simulink model "Template"  (Simulink 7.3)
settings: Solver=ode45  StartTime=0.0  StopTime=10.0  RelTol=1e-3
undefined symbols (not defined in the file): eta1_0_real, v1_0_real, velocitySatValues1
libraries: dspmtrx3 x21, simulink x14, dspindex x5, marine_gnc x4, simulink_extras x1, dspinverses x1
(part 2 of 4)

== system Template/Main Subsystems/Control/LgV2/alpha^q ==
  Add : Sum  OutDataType=fixdt(1, 16)  OutScaling=2^-10
  Add2 : Sum  OutDataType=fixdt(1, 16)  OutScaling=2^-10
  Add3 : Sum  OutDataType=fixdt(1, 16)  OutScaling=2^-10
  I : dspmtrx3/Constant Diagonal Matrix  SystemSampleTime=-1  q=[1 1 1 ]  frame=off  dataType=Inherit from 'Constant(s) along diagonal'  isSigned=on  wordLen=16  udDataType=sfix(16)  fracBitsMode=Best precision  numFracBits=15
  Product1 : Product  OutDataType=fixdt(1, 16)  OutScaling=2^0  RndMeth=Zero
  Product3 : Product  Inputs=3  Multiplication=Matrix(*)  OutDataType=fixdt(1, 16)  OutScaling=2^0  RndMeth=Zero
  Product4 : Product  Multiplication=Matrix(*)  OutDataType=fixdt(1, 16)  OutScaling=2^0  RndMeth=Zero
  tag scope: alpha__q=global
  wires:
  Add3/1 -> [alpha__q]
  Product1/1 -> Add/2
  [LgV2_kappa_1] -> Product1/1
  I/1 -> Product1/2
  Add/1 -> Product3/1
  Add2/1 -> Product4/2
  [R_psi__T] -> Product3/2, Product4/1
  [chi__q] -> Product3/3
  Product3/1 -> Add3/1
  Product4/1 -> Add3/2
  [LgV2_K_p] -> Add/1
  [g_q__q] -> Add2/1
  [g_s__q] -> Add2/2

== system Template/Main Subsystems/Control/LgV2/alpha^s ==
  Add1 : Sum  OutDataType=fixdt(1, 16)  OutScaling=2^-10
  Add2 : Sum  OutDataType=fixdt(1, 16)  OutScaling=2^-10
  Add3 : Sum  OutDataType=fixdt(1, 16)  OutScaling=2^-10
  I : dspmtrx3/Constant Diagonal Matrix  SystemSampleTime=-1  q=[1 1 1 ]  frame=off  dataType=Inherit from 'Constant(s) along diagonal'  isSigned=on  wordLen=16  udDataType=sfix(16)  fracBitsMode=Best precision  numFracBits=15
  Product1 : Product  OutDataType=fixdt(1, 16)  OutScaling=2^0  RndMeth=Zero
  Product3 : Product  Inputs=3  Multiplication=Matrix(*)  OutDataType=fixdt(1, 16)  OutScaling=2^0  RndMeth=Zero
  Product4 : Product  Multiplication=Matrix(*)  OutDataType=fixdt(1, 16)  OutScaling=2^0  RndMeth=Zero
  tag scope: alpha__s=global
  wires:
  Add3/1 -> [alpha__s]
  Product1/1 -> Add1/2
  [LgV2_kappa_1] -> Product1/1
  I/1 -> Product1/2
  Add1/1 -> Product3/1
  Add2/1 -> Product4/2
  [R_psi__T] -> Product3/2, Product4/1
  [chi__s] -> Product3/3
  Product3/1 -> Add3/1
  Product4/1 -> Add3/2
  [LgV2_K_p] -> Add1/1
  [g_q__s] -> Add2/1
  [g_s__s] -> Add2/2

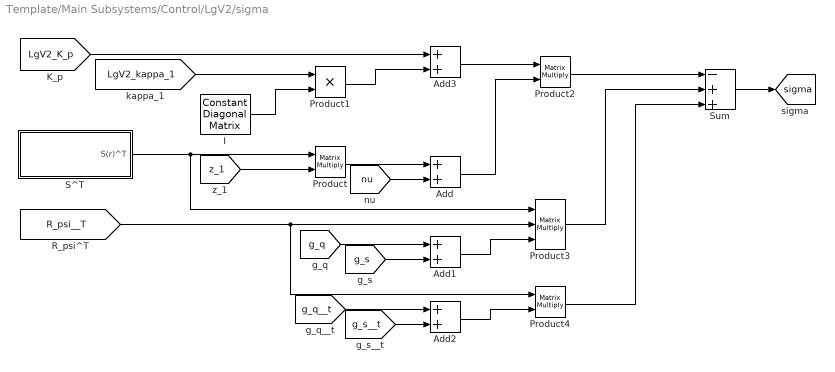
== system Template/Main Subsystems/Control/LgV2/sigma ==
  Add{,1..3} (4 alike) : Sum  OutDataType=fixdt(1, 16)  OutScaling=2^-10
  I : dspmtrx3/Constant Diagonal Matrix  SystemSampleTime=-1  q=[1 1 1 ]  frame=off  dataType=Inherit from 'Constant(s) along diagonal'  isSigned=on  wordLen=16  udDataType=sfix(16)  fracBitsMode=Best precision  numFracBits=15
  Product : Product  Multiplication=Matrix(*)  OutDataType=fixdt(1, 16)  OutScaling=2^0  RndMeth=Zero
  Product1 : Product  OutDataType=fixdt(1, 16)  OutScaling=2^0  RndMeth=Zero
  Product2 : Product  Multiplication=Matrix(*)  OutDataType=fixdt(1, 16)  OutScaling=2^0  RndMeth=Zero
  Product3 : Product  Inputs=3  Multiplication=Matrix(*)  OutDataType=fixdt(1, 16)  OutScaling=2^0  RndMeth=Zero
  Product4 : Product  Multiplication=Matrix(*)  OutDataType=fixdt(1, 16)  OutScaling=2^0  RndMeth=Zero
  S^T : Subsystem
  Sum : Sum  Inputs=-++  OutDataType=fixdt(1, 16)  OutScaling=2^-10
  tag scope: sigma=global
  wires:
  Sum/1 -> [sigma]
  [LgV2_K_p] -> Add3/1
  Product1/1 -> Add3/2
  [LgV2_kappa_1] -> Product1/1
  I/1 -> Product1/2
  S^T/1(S(r)^T) -> Product/1, Product3/1
  [z_1] -> Product/2
  Product/1 -> Add/1
  [nu] -> Add/2
  Add3/1 -> Product2/1
  Add/1 -> Product2/2
  Product2/1 -> Sum/1
  [g_q] -> Add1/1
  [g_s] -> Add1/2
  [g_q__t] -> Add2/1
  [g_s__t] -> Add2/2
  [R_psi__T] -> Product3/2, Product4/1
  Add1/1 -> Product3/3
  Add2/1 -> Product4/2
  Product3/1 -> Sum/2
  Product4/1 -> Sum/3

== system Template/Main Subsystems/Control/LgV2/z_1 ==
  Heading to -pi/pi : Subsystem
  Heading to -pi/pi1 : Subsystem
  Product : Product  Multiplication=Matrix(*)  OutDataType=fixdt(1, 16)  OutScaling=2^0  RndMeth=Zero
  Subtract : Sum  Inputs=+-  OutDataType=fixdt(1, 16)  OutScaling=2^-10
  tag scope: z_1=global
  wires:
  Subtract/1 -> Heading to -pi/pi1/1(eta(3) [0 2pi])
  Product/1 -> [z_1]
  Heading to -pi/pi/1(eta(3) [-pi pi]) -> Subtract/1
  Heading to -pi/pi1/1(eta(3) [-pi pi]) -> Product/2
  [R_psi__T] -> Product/1
  [chi] -> Subtract/2
  [eta] -> Heading to -pi/pi/1(eta(3) [0 2pi])

== system Template/Main Subsystems/Control/LgV2/z_2 ==
  Subtract : Sum  Inputs=+-  OutDataType=fixdt(1, 16)  OutScaling=2^-10
  tag scope: z_2=global
  wires:
  [alpha] -> Subtract/2
  Subtract/1 -> [z_2]
  [nu] -> Subtract/1

== system Template/Main Subsystems/Control/LgV2/zeta ==
  Integrator : Integrator  InitialCondition=[0 0 0]'
  Product : Product  Multiplication=Matrix(*)  OutDataType=fixdt(1, 16)  OutScaling=2^0  RndMeth=Zero
  tag scope: zeta=global
  wires:
  [R_psi] -> Product/1
  [z_2] -> Product/2
  Integrator/1 -> [zeta]
  Product/1 -> Integrator/1

== system Template/Main Subsystems/Control/Thruster allocation/VSP030 BT040 ==
  f_act : Inport
  BT_power_limit : Constant  Value=0.4
  Mux1 : Mux  Inputs=3
  VSP_speeds : Constant  Value=0.3
  f_act to u_act : Subsystem
  TC : Outport  OutDataType=fixdt(1, 16)  OutScaling=2^0
  wires:
  Mux1/1 -> TC/1
  f_act/1 -> f_act to u_act/1(f_act)
  BT_power_limit/1 -> Mux1/2
  VSP_speeds/1 -> Mux1/3
  f_act to u_act/1(u_act) -> Mux1/1

== system Template/Main Subsystems/Control/Thruster allocation/tau to f_act ==
  tau : Inport
  Product : Product  Multiplication=Matrix(*)  OutDataType=fixdt(1, 16)  OutScaling=2^0  RndMeth=Zero
  Pseudoinverse : dspinverses/Pseudoinverse  wanterr=off
  f_act : Outport
  wires:
  [B] -> Pseudoinverse/1
  Pseudoinverse/1 -> Product/1
  tau/1 -> Product/2
  Product/1 -> f_act/1

== system Template/Main Subsystems/Guidance/Line-Of-Sight Path-Following/Heading ==
  Demux : Demux  Outputs=2
  Demux1 : Demux  Outputs=2
  Demux2 : Demux  Outputs=2
  psi_d eq : Subsystem
  psi_d^s eq : Subsystem
  psi_d^s^2 eq : Subsystem
  tag scope: psi_d=global, psi_d__s=global, psi_d__s__2=global
  wires:
  psi_d^s eq/3(den) -> psi_d^s^2 eq/2(den)
  psi_d^s eq/2(num) -> psi_d^s^2 eq/1(num)
  Demux2/2 -> psi_d^s^2 eq/8(y_d^s^3)
  Demux2/1 -> psi_d^s^2 eq/7(x_d^s^3)
  psi_d^s^2 eq/1(psi_d^s^2) -> [psi_d__s__2]
  [p_d__s__3] -> Demux2/1
  psi_d^s eq/1(psi_d^s) -> [psi_d__s]
  Demux1/2 -> psi_d^s^2 eq/6(y_d^s^2), psi_d^s eq/4(y_d^s^2)
  Demux1/1 -> psi_d^s^2 eq/5(x_d^s^2), psi_d^s eq/3(x_d^s^2)
  [p_d__s__2] -> Demux1/1
  [p_d__s] -> Demux/1
  Demux/2 -> psi_d^s^2 eq/4(y_d^s), psi_d^s eq/2(y_d^s), psi_d eq/2(y_d^s)
  Demux/1 -> psi_d^s^2 eq/3(x_d^s), psi_d^s eq/1(x_d^s), psi_d eq/1(x_d^s)
  psi_d eq/1(psi_d) -> [psi_d]

== system Template/Main Subsystems/Guidance/Line-Of-Sight Path-Following/Line-Of-Sight ==
  Dynamic LOS assigment for qdot : Subsystem
  Dynamic assigment for sdot : Subsystem
  Gradient update law for sdot : Subsystem
  LOS heading : Subsystem
  Position error signals : Subsystem
  Subtract : Sum  Inputs=+-  OutDataType=fixdt(1, 16)  OutScaling=2^-10
  Virtual Vessel : Subsystem
  tag scope: diff_q_p_d=global
  wires:
  Gradient update law for sdot/3(omega_s^s) -> Dynamic assigment for sdot/6(omega_s^s)
  Gradient update law for sdot/2(omega_s^q) -> Dynamic assigment for sdot/5(omega_s^q)
  Position error signals/4(epsilon_n^q) -> Dynamic assigment for sdot/1(epsilon_n^q), LOS heading/4(epsilon_n^q)
  Position error signals/3(epsilon_n^s^2) -> LOS heading/3(epsilon_n^s^2)
  Position error signals/2(epsilon_n^q^2) -> LOS heading/2(epsilon_n^q^2)
  Position error signals/1(epsilon_n^qs) -> LOS heading/1(epsilon_n^qs)
  Position error signals/5(epsilon_n^s) -> Dynamic assigment for sdot/2(epsilon_n^s), LOS heading/5(epsilon_n^s)
  Position error signals/6(epsilon_n) -> LOS heading/6(epsilon_n), Dynamic assigment for sdot/3(epsilon_n)
  Gradient update law for sdot/1(omega_s) -> Dynamic assigment for sdot/4(omega_s)
  Subtract/1 -> [diff_q_p_d]
  [q] -> Subtract/1
  [p_d] -> Subtract/2

== system Template/Main Subsystems/Guidance/Line-Of-Sight Path-Following/Path ==
  note: Path Selector == 1: Linear path
      | Path Selector == 0: Ellipse path
  Ellipse path : Subsystem
  Path Switch workaround + limiter : Subsystem
  Straight path : Subsystem

== system Template/Main Subsystems/Guidance/Line-Of-Sight Path-Following/Speed assigment ==
  Derivative : Derivative
  v_s eq : Subsystem
  v_s^s eq : Subsystem
  v_s^t eq : Subsystem
  tag scope: u_d__t=global, v_s=global, v_s__s=global, v_s__t=global
  wires:
  Derivative/1 -> v_s^t eq/2(u_d^t), [u_d__t]
  v_s^t eq/1(v_s^t) -> [v_s__t]
  [p_d__s__2] -> v_s^s eq/4(p_d^s^2)
  [p_d__s] -> v_s^s eq/3(p_d^s)
  v_s^s eq/1(v_s^s) -> [v_s__s]
  [u_d] -> Derivative/1, v_s^s eq/2(u_d), v_s eq/2(u_d)
  [abs_p_d__s] -> v_s eq/1(|p_d^s|), v_s^s eq/1(|p_d^s|), v_s^t eq/1(|p_d^s|)
  v_s eq/1(v_s) -> [v_s]

== system Template/Main Subsystems/Plant/CSE1/Bow Thruster ==
  Bow Thruster Direction u_5 : Inport
  Bow Thruster Power : Inport  Port=2
  Add : Sum  Inputs=+++
  BT_D_Gain1 : Gain  Gain=0.02
  BT_D_Gain2 : Gain  Gain=0.02
  BT_L_Gain1 : Gain  Gain=0.02
  BT_L_Gain2 : Gain  Gain=-0.02
  BT_Power_Offset1 : Constant  Value=0.05
  BT_Power_Offset2 : Constant  Value=0.05
  BT_Power_Offset3 : Constant  Value=0.05
  Constant : Constant  Value=0  OutDataType=fixdt(1, 16)  OutScaling=2^0
  Constant1 : Constant  Value=0  OutDataType=fixdt(1, 16)  OutScaling=2^0
  Neg : Gain  Gain=-1  ParameterDataType=fixdt(1, 16)  ParameterScaling=2^0  OutDataType=fixdt(1, 16)  OutScaling=2^0
  SIT PWM0 BT : S-Function  Priority=1  FunctionName=NI_SIT_IO  Parameters=width dtype portnum stime stype btype  EnableBusSupport=off  mask(SIT Outport){portnum=1, width=-1, stime=-1, dtype=auto, stype=auto, btype=0}
      mask prompts: portnum "Port number:"; width "Port dimensions (-1 for dynamically sized):"; stime "Sample time (-1 for inherited):"; dtype "Data type:"; stype "Signal type:"; btype "Block type:"
      mask help: Use this outport on any level of nested subsystems to allow the LabVIEW Simulation Interface Toolkit to map hardware to it.
      mask init:
      | NI_SIT_IO_init;
      settings: CopyFcn=NI_SIT_IO_callbacks(1);  DeleteFcn=NI_SIT_IO_callbacks(2);
      mask StyleString: edit,edit,edit,popup(auto|double|single|int8|uint8|int16|uint16|int32|uint32|boolean),popup(auto|real|complex),edit
      mask CallbackString: NI_SIT_IO_callbacks(3);|||NI_SIT_IO_callbacks(4);||
      mask TabNameString: Parameters,Parameters,Parameters,Parameters,Parameters,Parameters
      mask Display:
      | patch([-x x], [-y y], [.90980 .81960 .32156]);
      | plot([0 -x x 0], [rad -y y rad]);
      | fprintf('SIT%d', portnum);
  Saturation Dynamic : simulink/Discontinuities/Saturation Dynamic  SystemSampleTime=-1  OutMin=[]  OutMax=[]  OutDataTypeStr=Inherit: Same as second input  OutDataType=fixdt(1, 16)  OutScaling=2^-10  DoSatur=off
  Saturation Dynamic1 : simulink/Discontinuities/Saturation Dynamic  SystemSampleTime=-1  OutMin=[]  OutMax=[]  OutDataTypeStr=Inherit: Same as second input  OutDataType=fixdt(1, 16)  OutScaling=2^-10  DoSatur=off
  Saturation Dynamic2 : simulink/Discontinuities/Saturation Dynamic  SystemSampleTime=-1  OutMin=[]  OutMax=[]  OutDataTypeStr=Inherit: Same as second input  OutDataType=fixdt(1, 16)  OutScaling=2^-10  DoSatur=off
  Sum1 : Sum  Inputs=|++
  Sum2 : Sum  Inputs=|++
  Terminator : Terminator
  Terminator1 : Terminator
  wires:
  Bow Thruster Direction u_5/1 -> BT_D_Gain1/1, Saturation Dynamic1/2, BT_D_Gain2/1, Saturation Dynamic2/2
  BT_D_Gain1/1 -> Add/1
  BT_D_Gain2/1 -> Add/3
  BT_Power_Offset1/1 -> Add/2
  Add/1 -> Saturation Dynamic/2
  Bow Thruster Power/1 -> BT_L_Gain2/1, Saturation Dynamic2/1, BT_L_Gain1/1, Neg/1
  Sum1/1 -> Saturation Dynamic/1
  BT_L_Gain1/1 -> Sum1/1
  BT_L_Gain2/1 -> Sum2/1
  Sum2/1 -> Saturation Dynamic/3
  BT_Power_Offset2/1 -> Sum1/2
  BT_Power_Offset3/1 -> Sum2/2
  Saturation Dynamic/1 -> SIT PWM0 BT/1
  Saturation Dynamic2/1 -> Terminator1/1
  Saturation Dynamic1/1 -> Terminator/1
  Constant/1 -> Saturation Dynamic1/1
  Constant1/1 -> Saturation Dynamic2/3
  Neg/1 -> Saturation Dynamic1/3

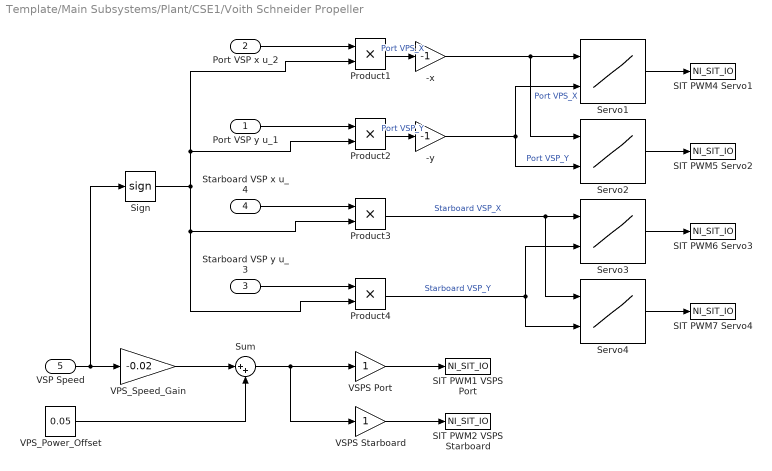
== system Template/Main Subsystems/Plant/CSE1/Voith Schneider Propeller  ==
  Port VSP y u_1 : Inport
  Port VSP x u_2 : Inport  Port=2
  Starboard VSP y u_3 : Inport  Port=3
  Starboard VSP x u_4 : Inport  Port=4
  VSP Speed : Inport  Port=5
  -x : Gain  Gain=-1
  -y : Gain  Gain=-1
  Product{1..4} (4 alike) : Product  RndMeth=Zero
  SIT PWM1 VSPS Port : S-Function  Priority=5  FunctionName=NI_SIT_IO  Parameters=width dtype portnum stime stype btype  EnableBusSupport=off  mask(SIT Outport){portnum=5, width=-1, stime=-1, dtype=auto, stype=auto, btype=0}
      mask prompts: portnum "Port number:"; width "Port dimensions (-1 for dynamically sized):"; stime "Sample time (-1 for inherited):"; dtype "Data type:"; stype "Signal type:"; btype "Block type:"
      mask help: Use this outport on any level of nested subsystems to allow the LabVIEW Simulation Interface Toolkit to map hardware to it.
      mask init:
      | NI_SIT_IO_init;
      settings: CopyFcn=NI_SIT_IO_callbacks(1);  DeleteFcn=NI_SIT_IO_callbacks(2);
      mask StyleString: edit,edit,edit,popup(auto|double|single|int8|uint8|int16|uint16|int32|uint32|boolean),popup(auto|real|complex),edit
      mask CallbackString: NI_SIT_IO_callbacks(3);|||NI_SIT_IO_callbacks(4);||
      mask TabNameString: Parameters,Parameters,Parameters,Parameters,Parameters,Parameters
      mask Display:
      | patch([-x x], [-y y], [.90980 .81960 .32156]);
      | plot([0 -x x 0], [rad -y y rad]);
      | fprintf('SIT%d', portnum);
  SIT PWM2 VSPS Starboard : S-Function  Priority=6  FunctionName=NI_SIT_IO  Parameters=width dtype portnum stime stype btype  EnableBusSupport=off  mask(SIT Outport){portnum=6, width=-1, stime=-1, dtype=auto, stype=auto, btype=0}
      mask prompts: portnum "Port number:"; width "Port dimensions (-1 for dynamically sized):"; stime "Sample time (-1 for inherited):"; dtype "Data type:"; stype "Signal type:"; btype "Block type:"
      mask help: Use this outport on any level of nested subsystems to allow the LabVIEW Simulation Interface Toolkit to map hardware to it.
      mask init:
      | NI_SIT_IO_init;
      settings: CopyFcn=NI_SIT_IO_callbacks(1);  DeleteFcn=NI_SIT_IO_callbacks(2);
      mask StyleString: edit,edit,edit,popup(auto|double|single|int8|uint8|int16|uint16|int32|uint32|boolean),popup(auto|real|complex),edit
      mask CallbackString: NI_SIT_IO_callbacks(3);|||NI_SIT_IO_callbacks(4);||
      mask TabNameString: Parameters,Parameters,Parameters,Parameters,Parameters,Parameters
      mask Display:
      | patch([-x x], [-y y], [.90980 .81960 .32156]);
      | plot([0 -x x 0], [rad -y y rad]);
      | fprintf('SIT%d', portnum);
  SIT PWM4 Servo1 : S-Function  Priority=1  FunctionName=NI_SIT_IO  Parameters=width dtype portnum stime stype btype  EnableBusSupport=off  mask(SIT Outport){portnum=1, width=-1, stime=-1, dtype=auto, stype=auto, btype=0}
      mask prompts: portnum "Port number:"; width "Port dimensions (-1 for dynamically sized):"; stime "Sample time (-1 for inherited):"; dtype "Data type:"; stype "Signal type:"; btype "Block type:"
      mask help: Use this outport on any level of nested subsystems to allow the LabVIEW Simulation Interface Toolkit to map hardware to it.
      mask init:
      | NI_SIT_IO_init;
      settings: CopyFcn=NI_SIT_IO_callbacks(1);  DeleteFcn=NI_SIT_IO_callbacks(2);
      mask StyleString: edit,edit,edit,popup(auto|double|single|int8|uint8|int16|uint16|int32|uint32|boolean),popup(auto|real|complex),edit
      mask CallbackString: NI_SIT_IO_callbacks(3);|||NI_SIT_IO_callbacks(4);||
      mask TabNameString: Parameters,Parameters,Parameters,Parameters,Parameters,Parameters
      mask Display:
      | patch([-x x], [-y y], [.90980 .81960 .32156]);
      | plot([0 -x x 0], [rad -y y rad]);
      | fprintf('SIT%d', portnum);
  SIT PWM5 Servo2 : S-Function  Priority=2  FunctionName=NI_SIT_IO  Parameters=width dtype portnum stime stype btype  EnableBusSupport=off  mask(SIT Outport){portnum=2, width=-1, stime=-1, dtype=auto, stype=auto, btype=0}
      mask prompts: portnum "Port number:"; width "Port dimensions (-1 for dynamically sized):"; stime "Sample time (-1 for inherited):"; dtype "Data type:"; stype "Signal type:"; btype "Block type:"
      mask help: Use this outport on any level of nested subsystems to allow the LabVIEW Simulation Interface Toolkit to map hardware to it.
      mask init:
      | NI_SIT_IO_init;
      settings: CopyFcn=NI_SIT_IO_callbacks(1);  DeleteFcn=NI_SIT_IO_callbacks(2);
      mask StyleString: edit,edit,edit,popup(auto|double|single|int8|uint8|int16|uint16|int32|uint32|boolean),popup(auto|real|complex),edit
      mask CallbackString: NI_SIT_IO_callbacks(3);|||NI_SIT_IO_callbacks(4);||
      mask TabNameString: Parameters,Parameters,Parameters,Parameters,Parameters,Parameters
      mask Display:
      | patch([-x x], [-y y], [.90980 .81960 .32156]);
      | plot([0 -x x 0], [rad -y y rad]);
      | fprintf('SIT%d', portnum);
  SIT PWM6 Servo3 : S-Function  Priority=3  FunctionName=NI_SIT_IO  Parameters=width dtype portnum stime stype btype  EnableBusSupport=off  mask(SIT Outport){portnum=3, width=-1, stime=-1, dtype=auto, stype=auto, btype=0}
      mask prompts: portnum "Port number:"; width "Port dimensions (-1 for dynamically sized):"; stime "Sample time (-1 for inherited):"; dtype "Data type:"; stype "Signal type:"; btype "Block type:"
      mask help: Use this outport on any level of nested subsystems to allow the LabVIEW Simulation Interface Toolkit to map hardware to it.
      mask init:
      | NI_SIT_IO_init;
      settings: CopyFcn=NI_SIT_IO_callbacks(1);  DeleteFcn=NI_SIT_IO_callbacks(2);
      mask StyleString: edit,edit,edit,popup(auto|double|single|int8|uint8|int16|uint16|int32|uint32|boolean),popup(auto|real|complex),edit
      mask CallbackString: NI_SIT_IO_callbacks(3);|||NI_SIT_IO_callbacks(4);||
      mask TabNameString: Parameters,Parameters,Parameters,Parameters,Parameters,Parameters
      mask Display:
      | patch([-x x], [-y y], [.90980 .81960 .32156]);
      | plot([0 -x x 0], [rad -y y rad]);
      | fprintf('SIT%d', portnum);
  SIT PWM7 Servo4 : S-Function  Priority=4  FunctionName=NI_SIT_IO  Parameters=width dtype portnum stime stype btype  EnableBusSupport=off  mask(SIT Outport){portnum=4, width=-1, stime=-1, dtype=auto, stype=auto, btype=0}
      mask prompts: portnum "Port number:"; width "Port dimensions (-1 for dynamically sized):"; stime "Sample time (-1 for inherited):"; dtype "Data type:"; stype "Signal type:"; btype "Block type:"
      mask help: Use this outport on any level of nested subsystems to allow the LabVIEW Simulation Interface Toolkit to map hardware to it.
      mask init:
      | NI_SIT_IO_init;
      settings: CopyFcn=NI_SIT_IO_callbacks(1);  DeleteFcn=NI_SIT_IO_callbacks(2);
      mask StyleString: edit,edit,edit,popup(auto|double|single|int8|uint8|int16|uint16|int32|uint32|boolean),popup(auto|real|complex),edit
      mask CallbackString: NI_SIT_IO_callbacks(3);|||NI_SIT_IO_callbacks(4);||
      mask TabNameString: Parameters,Parameters,Parameters,Parameters,Parameters,Parameters
      mask Display:
      | patch([-x x], [-y y], [.90980 .81960 .32156]);
      | plot([0 -x x 0], [rad -y y rad]);
      | fprintf('SIT%d', portnum);
  Servo1 : Lookup2D  RowIndex=[-1,0,1]  ColumnIndex=[-1,0,1]  Table=reshape([0.06,0.0495363,0.043301,0.06,0.052446,0.043301,0.06,0.0541518,0.043301],3,3)
  Servo2 : Lookup2D  RowIndex=[-1,0,1]  ColumnIndex=[-1,0,1]  Table=reshape([0.03860880,0.0386088,0.03860880,0.0459941,0.0477243,0.0500953,0.057,0.057,0.057],3,3)
  Servo3 : Lookup2D  RowIndex=[-1,0,1]  ColumnIndex=[-1,0,1]  Table=reshape([0.0640809,0.0640809,0.0640809,0.0539629,0.0541315,0.0556492,0.0442664,0.0442664,0.0442664],3,3)
  Servo4 : Lookup2D  RowIndex=[-1,0,1]  ColumnIndex=[-1,0,1]  Table=reshape([0.0602867,0.0470489,0.0403879,0.0602867,0.049747,0.0403879,0.0602867,0.0526138,0.0403879],3,3)
  Sign : Signum
  Sum : Sum  Inputs=|++
  VPS_Power_Offset : Constant  Value=0.05
  VPS_Speed_Gain : Gain  Gain=-0.02
  VSPS Port : Gain  ParameterDataType=fixdt(1, 16)  ParameterScaling=2^0  OutDataType=fixdt(1, 16)  OutScaling=2^0
  VSPS Starboard : Gain  ParameterDataType=fixdt(1, 16)  ParameterScaling=2^0  OutDataType=fixdt(1, 16)  OutScaling=2^0
  wires:
  Sign/1 -> Product1/2, Product2/2, Product3/2, Product4/2
  Product1/1 -> -x/1  "Port VPS_X"
  Product2/1 -> -y/1  "Port VSP_Y"
  Servo1/1 -> SIT PWM4 Servo1/1
  Servo2/1 -> SIT PWM5 Servo2/1
  Product3/1 -> Servo3/1, Servo4/1  "Starboard VSP_X"
  Product4/1 -> Servo3/2, Servo4/2  "Starboard VSP_Y"
  Servo3/1 -> SIT PWM6 Servo3/1
  Servo4/1 -> SIT PWM7 Servo4/1
  VSP Speed/1 -> VPS_Speed_Gain/1, Sign/1
  VPS_Speed_Gain/1 -> Sum/1
  VPS_Power_Offset/1 -> Sum/2
  Sum/1 -> VSPS Port/1, VSPS Starboard/1
  -y/1 -> Servo2/2, Servo1/2  "Port VSP_Y"
  -x/1 -> Servo1/1, Servo2/1  "Port VPS_X"
  Starboard VSP y u_3/1 -> Product4/1
  Starboard VSP x u_4/1 -> Product3/1
  Port VSP y u_1/1 -> Product2/1
  Port VSP x u_2/1 -> Product1/1
  VSPS Port/1 -> SIT PWM1 VSPS Port/1
  VSPS Starboard/1 -> SIT PWM2 VSPS Starboard/1

== system Template/Main Subsystems/Plant/Linear Simulator/Linear Vessel Dynamics ==
  note: This subsystem is a modifired version of Christoffer Throvaldsens Vessel Dynamic
  tau : Inport
  M_inv : Inport  Port=2
  D_L : Inport  Port=3
  Reset : Inport  Port=4
  eta_0 : Inport  Port=5
  nu_0 : Inport  Port=6
  Integrator : Integrator  ExternalReset=level  InitialConditionSource=external  InitialCondition=v1_0_real  UpperSaturationLimit=velocitySatValues1  LowerSaturationLimit=-1*velocitySatValues1
  Integrator1 : Integrator  ExternalReset=level  InitialConditionSource=external  InitialCondition=eta1_0_real
  Product1 : Product  Multiplication=Matrix(*)  RndMeth=Zero
  Product2 : Product  Multiplication=Matrix(*)  RndMeth=Zero
  Product3 : Product  Multiplication=Matrix(*)  RndMeth=Zero
  R(psi) : Subsystem
  Sum : Sum  Inputs=+-
  nudot : Terminator
  psi : Selector  InputPortWidth=3  IndexOptions=Index vector (dialog)  Indices=[3]  OutputSizes=1
  eta : Outport
  nu : Outport  Port=2
  etadot : Outport  Port=3
  wires:
  Sum/1 -> Product2/2
  Product2/1 -> Integrator/1, nudot/1
  Integrator/1 -> Product1/2, nu/1, Product3/2
  R(psi)/1(R) -> Product3/1
  psi/1 -> R(psi)/1(psi)
  M_inv/1 -> Product2/1
  tau/1 -> Sum/1
  Product1/1 -> Sum/2
  Product3/1 -> etadot/1, Integrator1/1
  Integrator1/1 -> psi/1, eta/1
  nu_0/1 -> Integrator/3
  Reset/1 -> Integrator/2, Integrator1/2
  eta_0/1 -> Integrator1/3
  D_L/1 -> Product1/1

== system Template/Main Subsystems/Control/LgV2/Auxilary functions g_q/g_q eq ==
  f_q : Inport
  psi_los^q : Inport  Port=2
  Product : Product  Multiplication=Matrix(*)  OutDataType=fixdt(1, 16)  OutScaling=2^0  RndMeth=Zero
  Vector Concatenate : Concatenate  Mode=Vector
  g_q : Outport
  wires:
  Vector Concatenate/1 -> g_q/1
  f_q/1 -> Vector Concatenate/1, Product/2
  psi_los^q/1 -> Product/1
  Product/1 -> Vector Concatenate/2

== system Template/Main Subsystems/Control/LgV2/Auxilary functions g_q/g_q^q eq ==
  f_q : Inport
  psi_los^q : Inport  Port=2
  f_q^q : Inport  Port=3
  psi_los^q^2 : Inport  Port=4
  Add : Sum  OutDataType=fixdt(1, 16)  OutScaling=2^-10
  Matrix Concatenate : Concatenate  Mode=Multidimensional array
  Product : Product  Multiplication=Matrix(*)  OutDataType=fixdt(1, 16)  OutScaling=2^0  RndMeth=Zero
  Product1 : Product  Multiplication=Matrix(*)  OutDataType=fixdt(1, 16)  OutScaling=2^0  RndMeth=Zero
  f_q^T : dspmtrx3/Transpose  SystemSampleTime=-1  Hermitian=off  overflowFlag=off
  psi_los^q^2T : dspmtrx3/Transpose  SystemSampleTime=-1  Hermitian=off  overflowFlag=off
  g_q^q : Outport
  wires:
  f_q^q/1 -> Matrix Concatenate/1, Product1/2
  Matrix Concatenate/1 -> g_q^q/1
  Add/1 -> Matrix Concatenate/2
  f_q/1 -> f_q^T/1
  f_q^T/1 -> Product/1
  psi_los^q^2/1 -> psi_los^q^2T/1
  Product/1 -> Add/1
  psi_los^q/1 -> Product1/1
  Product1/1 -> Add/2
  psi_los^q^2T/1 -> Product/2

== system Template/Main Subsystems/Control/LgV2/Auxilary functions g_q/g_q^s eq ==
  f_q : Inport
  psi_los^q : Inport  Port=2
  f_q^s : Inport  Port=3
  psi_los^qs : Inport  Port=4
  Add : Sum  OutDataType=fixdt(1, 16)  OutScaling=2^-10
  Product : Product  Multiplication=Matrix(*)  OutDataType=fixdt(1, 16)  OutScaling=2^0  RndMeth=Zero
  Product1 : Product  Multiplication=Matrix(*)  OutDataType=fixdt(1, 16)  OutScaling=2^0  RndMeth=Zero
  Vector Concatenate : Concatenate  Mode=Vector
  g_q^s : Outport
  wires:
  f_q^s/1 -> Vector Concatenate/1, Product1/2
  Vector Concatenate/1 -> g_q^s/1
  Add/1 -> Vector Concatenate/2
  Product/1 -> Add/1
  psi_los^q/1 -> Product1/1
  Product1/1 -> Add/2
  psi_los^qs/1 -> Product/1
  f_q/1 -> Product/2

== system Template/Main Subsystems/Control/LgV2/Auxilary functions g_q/g_q^t eq ==
  psi_los^q : Inport
  f_q^t : Inport  Port=2
  Product1 : Product  Multiplication=Matrix(*)  OutDataType=fixdt(1, 16)  OutScaling=2^0  RndMeth=Zero
  Vector Concatenate : Concatenate  Mode=Vector
  g_q^t : Outport
  wires:
  f_q^t/1 -> Vector Concatenate/1, Product1/2
  Vector Concatenate/1 -> g_q^t/1
  Product1/1 -> Vector Concatenate/2
  psi_los^q/1 -> Product1/1

== system Template/Main Subsystems/Control/LgV2/Auxiliary function g_s/g_s eq ==
  f_s : Inport
  psi_los^s : Inport  Port=2
  0_2x1 : Constant  Value=[0;0]  VectorParams1D=off  OutDataType=fixdt(1, 16)  OutScaling=2^0
  Product : Product  Multiplication=Matrix(*)  OutDataType=fixdt(1, 16)  OutScaling=2^0  RndMeth=Zero
  Vector Concatenate : Concatenate  Mode=Vector
  g_s : Outport
  wires:
  Vector Concatenate/1 -> g_s/1
  f_s/1 -> Product/2
  psi_los^s/1 -> Product/1
  Product/1 -> Vector Concatenate/2
  0_2x1/1 -> Vector Concatenate/1

== system Template/Main Subsystems/Control/LgV2/Auxiliary function g_s/g_s^q eq ==
  f_s : Inport
  psi_los^s : Inport  Port=2
  f_s^q : Inport  Port=3
  psi_los^sq : Inport  Port=4
  0_2x2 : Constant  Value=[0 0; 0 0]  VectorParams1D=off  OutDataType=fixdt(1, 16)  OutScaling=2^0
  Add : Sum  OutDataType=fixdt(1, 16)  OutScaling=2^-10
  Matrix Concatenate : Concatenate  Mode=Multidimensional array
  Product : Product  OutDataType=fixdt(1, 16)  OutScaling=2^0  RndMeth=Zero
  Product1 : Product  OutDataType=fixdt(1, 16)  OutScaling=2^0  RndMeth=Zero
  g_s^q : Outport
  wires:
  Matrix Concatenate/1 -> g_s^q/1
  Add/1 -> Matrix Concatenate/2
  Product/1 -> Add/1
  psi_los^s/1 -> Product1/1
  Product1/1 -> Add/2
  0_2x2/1 -> Matrix Concatenate/1
  f_s^q/1 -> Product1/2
  psi_los^sq/1 -> Product/1
  f_s/1 -> Product/2

== system Template/Main Subsystems/Control/LgV2/Auxiliary function g_s/g_s^s eq ==
  f_s : Inport
  psi_los^s : Inport  Port=2
  f_s^s : Inport  Port=3
  psi_los^s^2 : Inport  Port=4
  0_2x1 : Constant  Value=[0;0]  VectorParams1D=off  OutDataType=fixdt(1, 16)  OutScaling=2^0
  Add : Sum  OutDataType=fixdt(1, 16)  OutScaling=2^-10
  Product : Product  OutDataType=fixdt(1, 16)  OutScaling=2^0  RndMeth=Zero
  Product1 : Product  OutDataType=fixdt(1, 16)  OutScaling=2^0  RndMeth=Zero
  Vector Concatenate : Concatenate  Mode=Vector
  g_s^s : Outport
  wires:
  Vector Concatenate/1 -> g_s^s/1
  Add/1 -> Vector Concatenate/2
  Product/1 -> Add/1
  psi_los^s/1 -> Product1/1
  Product1/1 -> Add/2
  psi_los^s^2/1 -> Product/1
  f_s/1 -> Product/2
  0_2x1/1 -> Vector Concatenate/1
  f_s^s/1 -> Product1/2

== system Template/Main Subsystems/Control/LgV2/Auxiliary function g_s/g_s^t eq ==
  psi_los^s : Inport
  f_s^t : Inport  Port=2
  0_2x1 : Constant  Value=[0;0]  VectorParams1D=off  OutDataType=fixdt(1, 16)  OutScaling=2^0
  Product1 : Product  Multiplication=Matrix(*)  OutDataType=fixdt(1, 16)  OutScaling=2^0  RndMeth=Zero
  Vector Concatenate : Concatenate  Mode=Vector
  g_a^t : Outport
  wires:
  Vector Concatenate/1 -> g_a^t/1
  Product1/1 -> Vector Concatenate/2
  psi_los^s/1 -> Product1/1
  0_2x1/1 -> Vector Concatenate/1
  f_s^t/1 -> Product1/2

== system Template/Main Subsystems/Control/LgV2/sigma/S^T ==
  S(r) : Subsystem
  S^T : dspmtrx3/Transpose  SystemSampleTime=-1  Hermitian=off  overflowFlag=off
  r : Selector  InputPortWidth=3  IndexOptions=Index vector (dialog)  Indices=[3]  OutputSizes=1
  S(r)^T : Outport
  wires:
  r/1 -> S(r)/1(r)
  S(r)/1(S) -> S^T/1
  [nu] -> r/1
  S^T/1 -> S(r)^T/1

== system Template/Main Subsystems/Control/LgV2/z_1/Heading to -pi/pi ==
  eta(3) [0 2pi] : Inport
  Demux : Demux  Outputs=3
  Mux : Mux  Inputs=3
  rad to [-pi pi] : Subsystem
      mask Type: rad to pi/pi
      mask Description: Converts an angle in rad to between -pi and pi
      mask Display: disp('[0 2pi] to [-pi pi]')
  eta(3) [-pi pi] : Outport
  wires:
  Demux/3 -> rad to [-pi pi]/1(rad)
  Demux/1 -> Mux/1
  Demux/2 -> Mux/2
  eta(3) [0 2pi]/1 -> Demux/1
  Mux/1 -> eta(3) [-pi pi]/1
  rad to [-pi pi]/1("[-pi pi]") -> Mux/3

== system Template/Main Subsystems/Control/LgV2/z_1/Heading to -pi/pi1 ==
  eta(3) [0 2pi] : Inport
  Demux : Demux  Outputs=3
  Mux : Mux  Inputs=3
  rad to [-pi pi] : Subsystem
      mask Type: rad to pi/pi
      mask Description: Converts an angle in rad to between -pi and pi
      mask Display: disp('[0 2pi] to [-pi pi]')
  eta(3) [-pi pi] : Outport
  wires:
  rad to [-pi pi]/1("[-pi pi]") -> Mux/3
  Mux/1 -> eta(3) [-pi pi]/1
  eta(3) [0 2pi]/1 -> Demux/1
  Demux/2 -> Mux/2
  Demux/1 -> Mux/1
  Demux/3 -> rad to [-pi pi]/1(rad)

== system Template/Main Subsystems/Control/Thruster allocation/VSP030 BT040/f_act to u_act ==
  f_act : Inport
  Demux : Demux  Outputs=5
  Mux : Mux  Inputs=5
  f_1 to u_1 VSP speed 0.3 : Subsystem
  f_2 to u_2 VSP speed 0.3 : Subsystem
  f_3 to u_3 VSP speed 0.3 : Subsystem
  f_4 to u_4 VSP speed 0.3 : Subsystem
  f_5 to u_5 BT power 0.4 : Subsystem
  u_act : Outport
  wires:
  f_5 to u_5 BT power 0.4/1(u_5) -> Mux/5
  f_4 to u_4 VSP speed 0.3/1(u_4) -> Mux/4
  f_3 to u_3 VSP speed 0.3/1(u_3) -> Mux/3
  f_2 to u_2 VSP speed 0.3/1(u_2) -> Mux/2
  f_1 to u_1 VSP speed 0.3/1(u_1) -> Mux/1
  Demux/5 -> f_5 to u_5 BT power 0.4/1(f_5)
  Demux/4 -> f_4 to u_4 VSP speed 0.3/1(f_4)
  Demux/3 -> f_3 to u_3 VSP speed 0.3/1(f_3)
  Demux/1 -> f_1 to u_1 VSP speed 0.3/1(f_1)
  Mux/1 -> u_act/1
  f_act/1 -> Demux/1
  Demux/2 -> f_2 to u_2 VSP speed 0.3/1(f_2)

== system Template/Main Subsystems/Guidance/Line-Of-Sight Path-Following/Heading/psi_d eq ==
  x_d^s : Inport
  y_d^s : Inport  Port=2
  Trigonometric Function : Trigonometry  Operator=atan2
  rad to [-pi pi] : Subsystem
      mask Type: rad to pi/pi
      mask Description: Converts an angle in rad to between -pi and pi
      mask Display: disp('[0 2pi] to [-pi pi]')
  psi_d : Outport
  wires:
  x_d^s/1 -> Trigonometric Function/2
  y_d^s/1 -> Trigonometric Function/1
  rad to [-pi pi]/1("[-pi pi]") -> psi_d/1
  Trigonometric Function/1 -> rad to [-pi pi]/1(rad)

== system Template/Main Subsystems/Guidance/Line-Of-Sight Path-Following/Heading/psi_d^s eq ==
  x_d^s : Inport
  y_d^s : Inport  Port=2
  x_d^s^2 : Inport  Port=3
  y_d^s^2 : Inport  Port=4
  ( x_d^s )^2 : Math  Operator=square  OutDataType=fixdt(1, 16)  OutScaling=2^0  SaturateOnIntegerOverflow=on
  ( x_d^s )^2 + ( y_d^s )^2 : Sum  OutDataType=fixdt(1, 16)  OutScaling=2^-10
  "( x_d^s * y_d^s^2 ) - ( x_d^s^2 * y_d^s ) " : Sum  Inputs=+-  OutDataType=fixdt(1, 16)  OutScaling=2^-10
  ( y_d^s )^2 : Math  Operator=square  OutDataType=fixdt(1, 16)  OutScaling=2^0  SaturateOnIntegerOverflow=on
  Divide : Product  Inputs=*/  OutDataType=fixdt(1, 16)  OutScaling=2^-10
  x_d^s * y_d^s^2 : Product  OutDataType=fixdt(1, 16)  OutScaling=2^0  RndMeth=Zero
  x_d^s^2 * y_d^s : Product  OutDataType=fixdt(1, 16)  OutScaling=2^0  RndMeth=Zero
  psi_d^s : Outport
  num : Outport  Port=2
  den : Outport  Port=3
  wires:
  Divide/1 -> psi_d^s/1
  ( x_d^s )^2 + ( y_d^s )^2/1 -> den/1, Divide/2
  "( x_d^s * y_d^s^2 ) - ( x_d^s^2 * y_d^s ) "/1 -> num/1, Divide/1
  ( y_d^s )^2/1 -> ( x_d^s )^2 + ( y_d^s )^2/2
  ( x_d^s )^2/1 -> ( x_d^s )^2 + ( y_d^s )^2/1
  x_d^s^2 * y_d^s/1 -> "( x_d^s * y_d^s^2 ) - ( x_d^s^2 * y_d^s ) "/2
  x_d^s * y_d^s^2/1 -> "( x_d^s * y_d^s^2 ) - ( x_d^s^2 * y_d^s ) "/1
  x_d^s^2/1 -> x_d^s^2 * y_d^s/1
  y_d^s^2/1 -> x_d^s * y_d^s^2/2
  y_d^s/1 -> x_d^s^2 * y_d^s/2, ( y_d^s )^2/1
  x_d^s/1 -> x_d^s * y_d^s^2/1, ( x_d^s )^2/1

== system Template/Main Subsystems/Guidance/Line-Of-Sight Path-Following/Heading/psi_d^s^2 eq ==
  num : Inport
  den : Inport  Port=2
  x_d^s : Inport  Port=3
  y_d^s : Inport  Port=4
  x_d^s^2 : Inport  Port=5
  y_d^s^2 : Inport  Port=6
  x_d^s^3 : Inport  Port=7
  y_d^s^3 : Inport  Port=8
  ( x_d^s * x_d^s^2 ) + ( x_d^s^3 * y_d^s ) : Sum  OutDataType=fixdt(1, 16)  OutScaling=2^-10
  ( x_d^s * y_d^s^3  ) - ( x_d^s^3 * y_d^s ) : Sum  Inputs=+-  OutDataType=fixdt(1, 16)  OutScaling=2^-10
  * 2 : Gain  Gain=2  ParameterDataType=fixdt(1, 16)  ParameterScaling=2^0  OutDataType=fixdt(1, 16)  OutScaling=2^0
  Divide : Product  Inputs=*/  OutDataType=fixdt(1, 16)  OutScaling=2^-10
  Product1 : Product  OutDataType=fixdt(1, 16)  OutScaling=2^0  RndMeth=Zero
  Product2 : Product  OutDataType=fixdt(1, 16)  OutScaling=2^0  RndMeth=Zero
  Subtract : Sum  Inputs=+-  OutDataType=fixdt(1, 16)  OutScaling=2^-10
  "[ ( x_d^s )^2 + ( y_d^s )^2 ]^2" : Math  Operator=square  OutDataType=fixdt(1, 16)  OutScaling=2^0  SaturateOnIntegerOverflow=on
  x_d^s * x_d^s^2 : Product  OutDataType=fixdt(1, 16)  OutScaling=2^0  RndMeth=Zero
  "x_d^s * y_d^s^3 " : Product  OutDataType=fixdt(1, 16)  OutScaling=2^0  RndMeth=Zero
  x_d^s^3 * y_d^s : Product  OutDataType=fixdt(1, 16)  OutScaling=2^0  RndMeth=Zero
  y_d^s * y_d^s^2 : Product  OutDataType=fixdt(1, 16)  OutScaling=2^0  RndMeth=Zero
  psi_d^s^2 : Outport
  wires:
  Divide/1 -> psi_d^s^2/1
  "[ ( x_d^s )^2 + ( y_d^s )^2 ]^2"/1 -> Divide/2
  Subtract/1 -> Divide/1
  Product2/1 -> Subtract/2
  * 2/1 -> Product2/2
  ( x_d^s * x_d^s^2 ) + ( x_d^s^3 * y_d^s )/1 -> * 2/1
  num/1 -> Product2/1
  y_d^s^2/1 -> y_d^s * y_d^s^2/2
  y_d^s * y_d^s^2/1 -> ( x_d^s * x_d^s^2 ) + ( x_d^s^3 * y_d^s )/2
  x_d^s * x_d^s^2/1 -> ( x_d^s * x_d^s^2 ) + ( x_d^s^3 * y_d^s )/1
  x_d^s^2/1 -> x_d^s * x_d^s^2/2
  Product1/1 -> Subtract/1
  den/1 -> "[ ( x_d^s )^2 + ( y_d^s )^2 ]^2"/1, Product1/2
  ( x_d^s * y_d^s^3  ) - ( x_d^s^3 * y_d^s )/1 -> Product1/1
  x_d^s^3 * y_d^s/1 -> ( x_d^s * y_d^s^3  ) - ( x_d^s^3 * y_d^s )/2
  "x_d^s * y_d^s^3 "/1 -> ( x_d^s * y_d^s^3  ) - ( x_d^s^3 * y_d^s )/1
  y_d^s/1 -> y_d^s * y_d^s^2/1, x_d^s^3 * y_d^s/2
  x_d^s^3/1 -> x_d^s^3 * y_d^s/1
  y_d^s^3/1 -> "x_d^s * y_d^s^3 "/2
  x_d^s/1 -> x_d^s * x_d^s^2/1, "x_d^s * y_d^s^3 "/1

== system Template/Main Subsystems/Guidance/Line-Of-Sight Path-Following/Line-Of-Sight/Dynamic LOS assigment for qdot ==
  f_q eq : Subsystem
  f_q^q eq : Subsystem
  f_q^s eq : Subsystem
  f_q^t eq : Subsystem
  tag scope: f_q=global, f_q__q=global, f_q__s=global, f_q__t=global
  wires:
  [u_d__t] -> f_q^t eq/2(u_d^t)
  f_q^t eq/1(f_q^t) -> [f_q__t]
  [psi_los__s] -> f_q^s eq/3(psi_los^s)
  f_q^s eq/1(f_q^s) -> [f_q__s]
  f_q^q eq/1("f_q^q ") -> [f_q__q]
  [psi_los__q] -> f_q^q eq/3(psi_los^q)
  f_q eq/1(f_q) -> [f_q]
  [u_d] -> f_q^s eq/2(u_d), f_q^q eq/2(u_d), f_q eq/2(u_d)
  [psi_los] -> f_q^t eq/1(psi_los), f_q^s eq/1(psi_los), f_q^q eq/1(psi_los), f_q eq/1(psi_los)

== system Template/Main Subsystems/Guidance/Line-Of-Sight Path-Following/Line-Of-Sight/Dynamic assigment for sdot ==
  epsilon_n^q : Inport
  epsilon_n^s : Inport  Port=2
  epsilon_n : Inport  Port=3
  omega_s : Inport  Port=4
  omega_s^q : Inport  Port=5
  omega_s^s : Inport  Port=6
  f_s eq : Subsystem
  f_s^q eq : Subsystem
  f_s^s eq : Subsystem
  f_s^t eq : Subsystem
  tag scope: f_s=global, f_s__q=global, f_s__s=global, f_s__t=global
  wires:
  [v_s__t] -> f_s^t eq/3(v_s^t)
  [v_s__s] -> f_s^s eq/6(v_s^s)
  epsilon_n^s/1 -> f_s^s eq/5(epsilon_n^s)
  omega_s^s/1 -> f_s^s eq/4(omega_s^s)
  epsilon_n^q/1 -> f_s^q eq/5(epsilon_n^q)
  omega_s^q/1 -> f_s^q eq/4(omega_s^q)
  omega_s/1 -> f_s eq/4(omega_s)
  [v_s] -> f_s^s eq/3(v_s), f_s^q eq/3(v_s), f_s eq/3(v_s)
  epsilon_n/1 -> f_s^t eq/2(epsilon_n), f_s^s eq/2(epsilon_n), f_s^q eq/2(epsilon_n), f_s eq/2(epsilon_n)
  [Delta] -> f_s^t eq/1(Delta), f_s^s eq/1(Delta), f_s^q eq/1(Delta), f_s eq/1(Delta)
  f_s eq/1(f_s) -> [f_s]
  f_s^q eq/1(f_s^q) -> [f_s__q]
  f_s^s eq/1(f_s^s) -> [f_s__s]
  f_s^t eq/1(f_s^t) -> [f_s__t]

== system Template/Main Subsystems/Guidance/Line-Of-Sight Path-Following/Line-Of-Sight/Gradient update law for sdot ==
  omega_s eq : Subsystem
  omega_s^q eq : Subsystem
  omega_s^s eq : Subsystem
  omega_s : Outport
  omega_s^q : Outport  Port=2
  omega_s^s : Outport  Port=3
  wires:
  [diff_q_p_d] -> omega_s^s eq/2(q - p_d), omega_s eq/2(q - p_d)
  omega_s^s eq/1(omega_s^s) -> omega_s^s/1
  omega_s^q eq/1(omega_s^q) -> omega_s^q/1
  omega_s eq/1(omega_s) -> omega_s/1
  [abs_p_d__s] -> omega_s eq/4(|p_d^s|), omega_s^s eq/4(|p_d^s|), omega_s^q eq/3(|p_d^s|)
  [Path_my] -> omega_s eq/3(my), omega_s^s eq/3(my), omega_s^q eq/2(my)
  [p_d__s] -> omega_s^s eq/1(p_d^s), omega_s^q eq/1(p_d^s), omega_s eq/1(p_d^s)
  [p_d__s__2] -> omega_s^s eq/5(p_d^s^2)

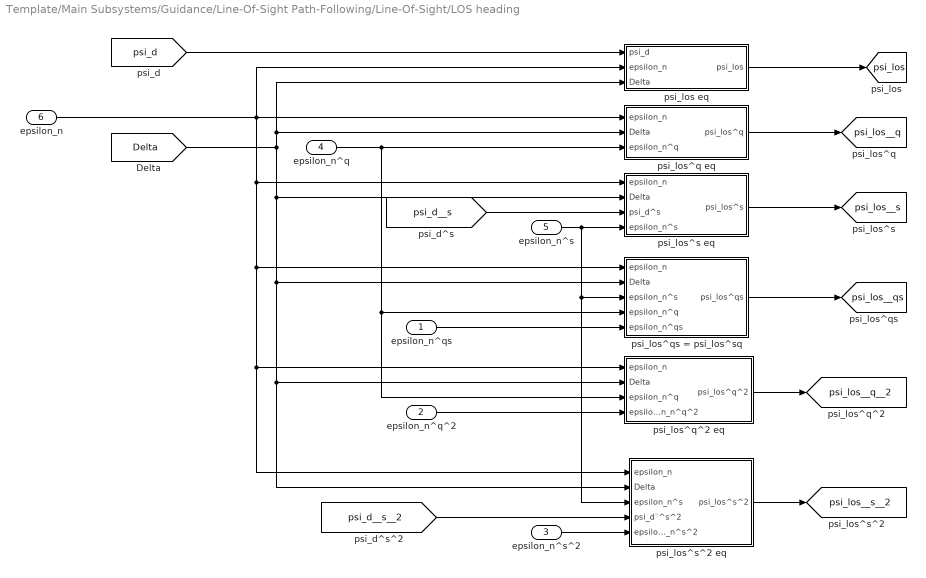
== system Template/Main Subsystems/Guidance/Line-Of-Sight Path-Following/Line-Of-Sight/LOS heading ==
  epsilon_n^qs : Inport
  epsilon_n^q^2 : Inport  Port=2
  epsilon_n^s^2 : Inport  Port=3
  epsilon_n^q : Inport  Port=4
  epsilon_n^s : Inport  Port=5
  epsilon_n : Inport  Port=6
  psi_los eq : Subsystem
  psi_los^q eq : Subsystem
  psi_los^q^2 eq : Subsystem
  psi_los^qs = psi_los^sq : Subsystem
  psi_los^s eq : Subsystem
  psi_los^s^2 eq : Subsystem
  tag scope: psi_los=global, psi_los__q=global, psi_los__q__2=global, psi_los__qs=global, psi_los__s=global, psi_los__s__2=global
  wires:
  psi_los^s^2 eq/1(psi_los^s^2) -> [psi_los__s__2]
  epsilon_n^s^2/1 -> psi_los^s^2 eq/5(epsilon_n^s^2)
  [psi_d__s__2] -> psi_los^s^2 eq/4(psi_d¨^s^2)
  epsilon_n^q^2/1 -> psi_los^q^2 eq/4(epsilon_n^q^2)
  psi_los^q^2 eq/1(psi_los^q^2) -> [psi_los__q__2]
  epsilon_n^qs/1 -> psi_los^qs = psi_los^sq/5(epsilon_n^qs)
  epsilon_n^s/1 -> psi_los^s eq/4(epsilon_n^s), psi_los^s^2 eq/3(epsilon_n^s), psi_los^qs = psi_los^sq/3(epsilon_n^s)
  psi_los^qs = psi_los^sq/1(psi_los^qs) -> [psi_los__qs]
  [psi_d__s] -> psi_los^s eq/3(psi_d^s)
  psi_los^s eq/1(psi_los^s) -> [psi_los__s]
  psi_los^q eq/1(psi_los^q) -> [psi_los__q]
  epsilon_n^q/1 -> psi_los^q eq/3(epsilon_n^q), psi_los^q^2 eq/3(epsilon_n^q), psi_los^qs = psi_los^sq/4(epsilon_n^q)
  [Delta] -> psi_los^q eq/2(Delta), psi_los^s eq/2(Delta), psi_los^qs = psi_los^sq/2(Delta), psi_los^s^2 eq/2(Delta), psi_los^q^2 eq/2(Delta), psi_los eq/3(Delta)
  epsilon_n/1 -> psi_los^q eq/1(epsilon_n), psi_los^s eq/1(epsilon_n), psi_los^qs = psi_los^sq/1(epsilon_n), psi_los^s^2 eq/1(epsilon_n), psi_los^q^2 eq/1(epsilon_n), psi_los eq/2(epsilon_n)
  [psi_d] -> psi_los eq/1(psi_d)
  psi_los eq/1(psi_los) -> [psi_los]

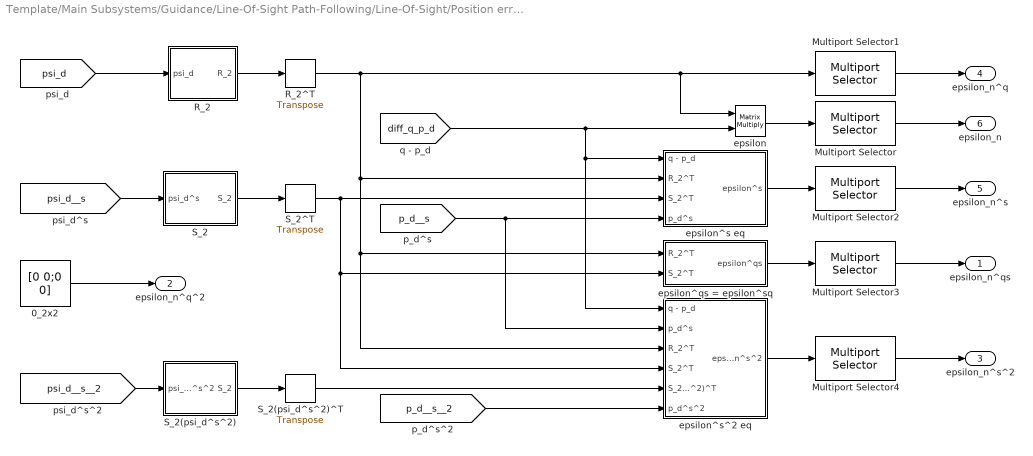
== system Template/Main Subsystems/Guidance/Line-Of-Sight Path-Following/Line-Of-Sight/Position error signals ==
  0_2x2 : Constant  Value=[0 0;0 0]  OutDataType=fixdt(1, 16)  OutScaling=2^0
  Multiport Selector{,1..4} (5 alike) : dspindex/Multiport Selector  rowsOrCols=Rows  idxCellArray={2}  idxErrMode=Clip Index
  R_2 : Subsystem  TreatAsAtomicUnit=on
      settings: MinAlgLoopOccurrences=on
  R_2^T : dspmtrx3/Transpose  SystemSampleTime=-1  Hermitian=off  overflowFlag=off
  S_2 : Subsystem  TreatAsAtomicUnit=on
      settings: MinAlgLoopOccurrences=on
  S_2(psi_d^s^2) : Subsystem  TreatAsAtomicUnit=on
      settings: MinAlgLoopOccurrences=on
  S_2(psi_d^s^2)^T : dspmtrx3/Transpose  SystemSampleTime=-1  Hermitian=off  overflowFlag=off
  S_2^T : dspmtrx3/Transpose  SystemSampleTime=-1  Hermitian=off  overflowFlag=off
  epsilon : Product  Multiplication=Matrix(*)  OutDataType=fixdt(1, 16)  OutScaling=2^0  RndMeth=Zero
  epsilon^qs = epsilon^sq : Subsystem
  epsilon^s eq : Subsystem
  epsilon^s^2 eq : Subsystem
  epsilon_n^qs : Outport
  epsilon_n^q^2 : Outport  Port=2
  epsilon_n^s^2 : Outport  Port=3
  epsilon_n^q : Outport  Port=4
  epsilon_n^s : Outport  Port=5
  epsilon_n : Outport  Port=6
  wires:
  Multiport Selector1/1 -> epsilon_n^q/1
  [p_d__s__2] -> epsilon^s^2 eq/6(p_d^s^2)
  S_2(psi_d^s^2)^T/1 -> epsilon^s^2 eq/5(S_2(psi_d^s^2)^T)
  Multiport Selector4/1 -> epsilon_n^s^2/1
  epsilon^s^2 eq/1(epsilon^s^2) -> Multiport Selector4/1
  S_2(psi_d^s^2)/1(S_2) -> S_2(psi_d^s^2)^T/1
  Multiport Selector3/1 -> epsilon_n^qs/1
  Multiport Selector2/1 -> epsilon_n^s/1
  Multiport Selector/1 -> epsilon_n/1
  epsilon/1 -> Multiport Selector/1
  0_2x2/1 -> epsilon_n^q^2/1
  epsilon^qs = epsilon^sq/1(epsilon^qs) -> Multiport Selector3/1
  S_2^T/1 -> epsilon^s^2 eq/4(S_2^T), epsilon^qs = epsilon^sq/2(S_2^T), epsilon^s eq/3(S_2^T)
  epsilon^s eq/1(epsilon^s) -> Multiport Selector2/1
  [p_d__s] -> epsilon^s^2 eq/2(p_d^s), epsilon^s eq/4(p_d^s)
  S_2/1(S_2) -> S_2^T/1
  [diff_q_p_d] -> epsilon^s^2 eq/1(q - p_d), epsilon^s eq/1(q - p_d), epsilon/2
  R_2^T/1 -> epsilon^s^2 eq/3(R_2^T), epsilon^qs = epsilon^sq/1(R_2^T), epsilon^s eq/2(R_2^T), Multiport Selector1/1, epsilon/1
  [psi_d] -> R_2/1(psi_d)
  R_2/1(R_2) -> R_2^T/1
  [psi_d__s] -> S_2/1(psi_d^s)
  [psi_d__s__2] -> S_2(psi_d^s^2)/1(psi_d^s^2)

== system Template/Main Subsystems/Guidance/Line-Of-Sight Path-Following/Line-Of-Sight/Virtual Vessel ==
  0_2x1 : Constant  Value=[0;0]  VectorParams1D=off  OutDataType=fixdt(1, 16)  OutScaling=2^0
  I : dspmtrx3/Constant Diagonal Matrix  SystemSampleTime=-1  q=[1 1]  frame=off  dataType=Inherit from 'Constant(s) along diagonal'  isSigned=on  wordLen=16  udDataType=sfix(16)  fracBitsMode=Best precision  numFracBits=15
  Matrix Concatenate : Concatenate  Mode=Multidimensional array
  Vector Concatenate : Concatenate  Mode=Vector
  Vector Concatenate1 : Concatenate  Mode=Vector
  tag scope: chi=global, chi__q=global, chi__s=global
  wires:
  0_2x1/1 -> Vector Concatenate1/1
  Vector Concatenate1/1 -> [chi__s]
  Matrix Concatenate/1 -> [chi__q]
  [psi_los__q] -> Matrix Concatenate/2
  I/1 -> Matrix Concatenate/1
  Vector Concatenate/1 -> [chi]
  [psi_los] -> Vector Concatenate/2
  [q] -> Vector Concatenate/1
  [psi_los__s] -> Vector Concatenate1/2

== system Template/Main Subsystems/Guidance/Line-Of-Sight Path-Following/Path/Ellipse path ==
  p_d eq : Subsystem
  p_d^s eq : Subsystem
  p_d^s^2 eq : Subsystem
  p_d^s^3 eq : Subsystem
  |p_d^s| eq : Subsystem
  tag scope: E_abs_p_d__s=global, E_p_d=global, E_p_d__s=global, E_p_d__s__2=global, E_p_d__s__3=global
  wires:
  p_d^s eq/1(p_d^s) -> [E_p_d__s], |p_d^s| eq/1(p_d^s)
  [s] -> p_d eq/1(s), p_d^s eq/1(s), p_d^s^2 eq/1(s), p_d^s^3 eq/1(s)
  [r_x] -> p_d eq/2(r_x), p_d^s eq/2(r_x), p_d^s^2 eq/2(r_x), p_d^s^3 eq/2(r_x)
  [r_y] -> p_d eq/3(r_y), p_d^s eq/3(r_y), p_d^s^2 eq/3(r_y), p_d^s^3 eq/3(r_y)
  [origin_x] -> p_d eq/4(origo_x)
  [origin_y] -> p_d eq/5(origo_y)
  [k] -> p_d eq/6(k), p_d^s eq/4(k), p_d^s^2 eq/4(k), p_d^s^3 eq/4(k)
  p_d eq/1(p_d) -> [E_p_d]
  |p_d^s| eq/1(|p_d^s|) -> [E_abs_p_d__s]
  p_d^s^2 eq/1(p_d^s^2) -> [E_p_d__s__2]
  p_d^s^3 eq/1(p_d^s^3) -> [E_p_d__s__3]

== system Template/Main Subsystems/Guidance/Line-Of-Sight Path-Following/Path/Path Switch workaround + limiter ==
  note: Path Selector == 1: Linear path
      | Path Selector == 0: Ellipse path
  Limiter : Subsystem
  p_d selcetor : Subsystem
  p_d^s selcetor : Subsystem
  p_d^s^2 selcetor : Subsystem
  p_d^s^3 selcetor : Subsystem
  p_d^s^3 selcetor1 : Subsystem
  tag scope: abs_p_d__s=global, p_d=global, p_d__s=global, p_d__s__2=global, p_d__s__3=global
  wires:
  [Path_Selector] -> p_d selcetor/1(Path Selector), p_d^s selcetor/1(Path Selector), p_d^s^2 selcetor/1(Path Selector), p_d^s^3 selcetor/1(Path Selector), p_d^s^3 selcetor1/1(Path Selector)  "chosen path"
  p_d selcetor/1(p_d) -> Limiter/1(p_d)
  Limiter/1(sat_p_d) -> [p_d]
  p_d^s selcetor/1(p_d^s) -> [p_d__s]
  p_d^s^2 selcetor/1(p_d^s^2) -> [p_d__s__2]
  p_d^s^3 selcetor/1(p_d^s^3) -> [p_d__s__3]
  p_d^s^3 selcetor1/1(|p_d^s|) -> [abs_p_d__s]

== system Template/Main Subsystems/Guidance/Line-Of-Sight Path-Following/Path/Straight path ==
  0_2x1 : Constant  Value=[0;0]  VectorParams1D=off  OutDataType=fixdt(1, 16)  OutScaling=2^0
  p_d eq : Subsystem
  p_d^s eq : Subsystem
  |p_d^s| eq : Subsystem
  tag scope: L_abs_p_d__s=global, L_p_d=global, L_p_d__s=global, L_p_d__s__2=global, L_p_d__s__3=global
  wires:
  p_d eq/1(p_d) -> [L_p_d]
  0_2x1/1 -> [L_p_d__s__2], [L_p_d__s__3]
  [y_2] -> p_d eq/5(y_2), p_d^s eq/4(y_2)
  [x_2] -> p_d eq/4(x_2), p_d^s eq/3(x_2)
  [y_1] -> p_d eq/3(y_1), p_d^s eq/2(y_1)
  [x_1] -> p_d eq/2(x_1), p_d^s eq/1(x_1)
  [s] -> p_d eq/1(s)
  |p_d^s| eq/1(|p_d^s|) -> [L_abs_p_d__s]
  p_d^s eq/1(p_d^s) -> |p_d^s| eq/1(p_d^s), [L_p_d__s]

== system Template/Main Subsystems/Guidance/Line-Of-Sight Path-Following/Speed assigment/v_s eq ==
  |p_d^s| : Inport
  u_d : Inport  Port=2
  Divide : Product  Inputs=*/  OutDataType=fixdt(1, 16)  OutScaling=2^-10
  v_s : Outport
  wires:
  |p_d^s|/1 -> Divide/2
  u_d/1 -> Divide/1
  Divide/1 -> v_s/1

== system Template/Main Subsystems/Guidance/Line-Of-Sight Path-Following/Speed assigment/v_s^s eq ==
  |p_d^s| : Inport
  u_d : Inport  Port=2
  p_d^s : Inport  Port=3
  p_d^s^2 : Inport  Port=4
  Constant : Constant  Value=3  OutDataType=fixdt(1, 16)  OutScaling=2^0
  Divide : Product  Inputs=*/  OutDataType=fixdt(1, 16)  OutScaling=2^-10
  Gain : Gain  Gain=-1  ParameterDataType=fixdt(1, 16)  ParameterScaling=2^0  OutDataType=fixdt(1, 16)  OutScaling=2^0
  Product : Product  OutDataType=fixdt(1, 16)  OutScaling=2^0  RndMeth=Zero
  Product1 : Product  Multiplication=Matrix(*)  OutDataType=fixdt(1, 16)  OutScaling=2^0  RndMeth=Zero
  p_d^s^T : dspmtrx3/Transpose  SystemSampleTime=-1  Hermitian=off  overflowFlag=off
  |p_d^s|^3 : Math  Operator=pow  OutDataType=fixdt(1, 16)  OutScaling=2^0  SaturateOnIntegerOverflow=on
  v_s^s : Outport
  wires:
  Gain/1 -> v_s^s/1
  u_d/1 -> Product/2
  Divide/1 -> Product/1
  |p_d^s|^3/1 -> Divide/2
  Product1/1 -> Divide/1
  Constant/1 -> |p_d^s|^3/2
  |p_d^s|/1 -> |p_d^s|^3/1
  p_d^s^2/1 -> Product1/2
  p_d^s^T/1 -> Product1/1
  p_d^s/1 -> p_d^s^T/1
  Product/1 -> Gain/1

== system Template/Main Subsystems/Guidance/Line-Of-Sight Path-Following/Speed assigment/v_s^t eq ==
  |p_d^s| : Inport
  u_d^t : Inport  Port=2
  Divide : Product  Inputs=*/  OutDataType=fixdt(1, 16)  OutScaling=2^-10
  v_s^t : Outport
  wires:
  |p_d^s|/1 -> Divide/2
  u_d^t/1 -> Divide/1
  Divide/1 -> v_s^t/1

== system Template/Main Subsystems/Plant/Linear Simulator/Linear Vessel Dynamics/R(psi) ==
  psi : Inport
  Mux : Mux  Inputs=9
  R(psi) : Reshape  OutputDimensionality=Customize  OutputDimensions=[3,3]
  R11 : Fcn  Expr=cos(u(1))
  R12 : Fcn  Expr=-1*sin(u(1))
  R{13,23,31..32} (4 alike) : Constant  Value=0
  R21 : Fcn  Expr=sin(u(1))
  R22 : Fcn  Expr=cos(u(1))
  R33 : Constant
  R : Outport
  wires:
  R(psi)/1 -> R/1
  Mux/1 -> R(psi)/1
  psi/1 -> R11/1, R21/1, R12/1, R22/1
  R11/1 -> Mux/1
  R21/1 -> Mux/2
  R31/1 -> Mux/3
  R12/1 -> Mux/4
  R22/1 -> Mux/5
  R32/1 -> Mux/6
  R13/1 -> Mux/7
  R33/1 -> Mux/9
  R23/1 -> Mux/8

== system Template/Main Subsystems/Control/LgV2/sigma/S^T/S(r) ==
  r : Inport
  Mux : Mux  Inputs=9
  R31 : Constant  Value=0
  S(r) : Reshape  OutputDimensionality=Customize  OutputDimensions=[3,3]
  S{11,13,22..23,32} (5 alike) : Constant  Value=0
  S12 : Gain  ParameterDataType=fixdt(1, 16)  ParameterScaling=2^0  OutDataType=fixdt(1, 16)  OutScaling=2^0
  S33 : Constant
  S : Outport
  wires:
  S(r)/1 -> S/1
  Mux/1 -> S(r)/1
  R31/1 -> Mux/3
  S12/1 -> Mux/4
  S22/1 -> Mux/5
  S32/1 -> Mux/6
  S13/1 -> Mux/7
  S33/1 -> Mux/9
  S23/1 -> Mux/8
  r/1 -> Mux/2, S12/1
  S11/1 -> Mux/1

== system Template/Main Subsystems/Control/LgV2/z_1/Heading to -pi/pi/rad to [-pi pi] ==
  rad : Inport  OutDataType=sfix(16)  OutScaling=2^0
  Constant : Constant  Value=2*pi  OutDataType=sfix(16)  OutScaling=2^0
  Gain : Gain  Gain=pi  ParameterDataType=sfix(16)  ParameterScaling=2^0  OutDataType=sfix(16)  OutScaling=2^0  SaturateOnIntegerOverflow=on  OutDataTypeStr=Inherit: Same as input  ParamDataTypeStr=Inherit: Same as input
  Math Function : Math  Operator=rem  OutDataType=sfix(16)  OutScaling=2^0  SaturateOnIntegerOverflow=on
  Saturation : Saturate  UpperLimit=1e10  LowerLimit=-1e10
  Sign : Signum
  Sum : Sum  Inputs=|+-  OutDataType=sfix(16)  OutScaling=2^0  SaturateOnIntegerOverflow=on
  Sum1 : Sum  Inputs=|++  OutDataType=sfix(16)  OutScaling=2^0  SaturateOnIntegerOverflow=on
  "[-pi pi]" : Outport  OutDataType=sfix(16)  OutScaling=2^0
  wires:
  Sum/1 -> "[-pi pi]"/1
  Math Function/1 -> Sum/1
  Constant/1 -> Math Function/2
  Sum1/1 -> Math Function/1
  Gain/1 -> Sum1/2, Sum/2
  Sign/1 -> Gain/1
  rad/1 -> Saturation/1
  Saturation/1 -> Sign/1, Sum1/1
